simulink model "einspurmodell"  (R2017a)
settings: Solver=ode5  StartTime=0.0  StopTime=t_final  FixedStep=delta_t  RelTol=1e-3  EnableMultiTasking=on
PreLoadFcn:
  | model_preload_function;
InitFcn:
  | model_init_function;
values from neighbouring files (symbols this model uses):
  A = 1.9    [model_preload_function.m]
  alpha_q0 = pq_1*pq_2 + pq_1*pq_3 + pq_2*pq_3    (= 135)    [model_preload_function.m]
  alpha_q1 = -1 * (pq_1 + pq_2 + pq_3)    (= 23)    [model_preload_function.m]
  alpha_q_ = -1 * pq_1 * pq_2 * pq_3    (= 225)    [model_preload_function.m]
  c_h = 100000    [model_preload_function.m]
  c_v = 100000    [model_preload_function.m]
  c_w = 0.28    [model_preload_function.m]
  kiv = pv_1*pv_2    (= 0.48)    [model_preload_function.m]
  kpv = -pv_1-pv_2    (= 4.9)    [model_preload_function.m]
  l_h = 1.45    [model_preload_function.m]
  l_l0 = 10    [model_preload_function.m]
  l_v = 1.3    [model_preload_function.m]
  m = 1450    [model_preload_function.m]
  psi_0 = 0    [model_preload_function.m]
  rho_luft = 1.204    [model_preload_function.m]
  theta = 1920    [model_preload_function.m]
  v_0 = 10    [model_preload_function.m]
  v_soll = 10    [model_preload_function.m]
  w_ltr = 0    [model_preload_function.m]
  x_0 = 00    (= 0)    [model_preload_function.m]
  y_0 = 1.5    [model_preload_function.m]
undefined symbols (not defined in the file or in its folder): Ap, Bp, Cp, Dp
libraries: simulink x1
settings Model: Creator=piwi  LastModifiedBy=hi
settings DataIOCC: LimitDataPoints=on  SaveFormat=Array  SignalLoggingSaveFormat=ModelDataLogs  SignalLoggingName=sigsOut
settings OptimizationCC: LifeSpan=inf
settings DebuggingCC: SaveWithParameterizedLinksMsg=none  UnderspecifiedInitializationDetection=Classic  MergeDetectMultiDrivingBlocksExec=none  SignalResolutionControl=TryResolveAllWithWarning  MultiTaskDSMMsg=warning  MultiTaskCondExecSysMsg=none  SFUnexpectedBacktrackingDiag=warning  SFNoUnconditionalDefaultTransitionDiag=warning  SFExecutionAtInitializationDiag=none
settings HardwareCC: ProdBitPerPointer=32  ProdBitPerSizeT=32  ProdBitPerPtrDiffT=32  ProdLargestAtomicFloat=None  ProdIntDivRoundTo=Undefined  ProdEndianess=Unspecified  ProdWordSize=32  ProdHWDeviceType=32-bit Generic  TargetUnknown=on
settings ModelReferenceCC: PropagateSignalLabelsOutOfModel=off
settings GRTTargetCC: TargetLangStandard=C89/C90 (ANSI)  GeneratePreprocessorConditionals=Disable all  CombineOutputUpdateFcns=off  GRTInterface=on
settings ConfigComp: CovMetricSettings=dw  CovHtmlReporting=on  CovSaveCumulativeToWorkspaceVar=on  CovSaveSingleToWorkspaceVar=on  CovExternalEMLEnable=off

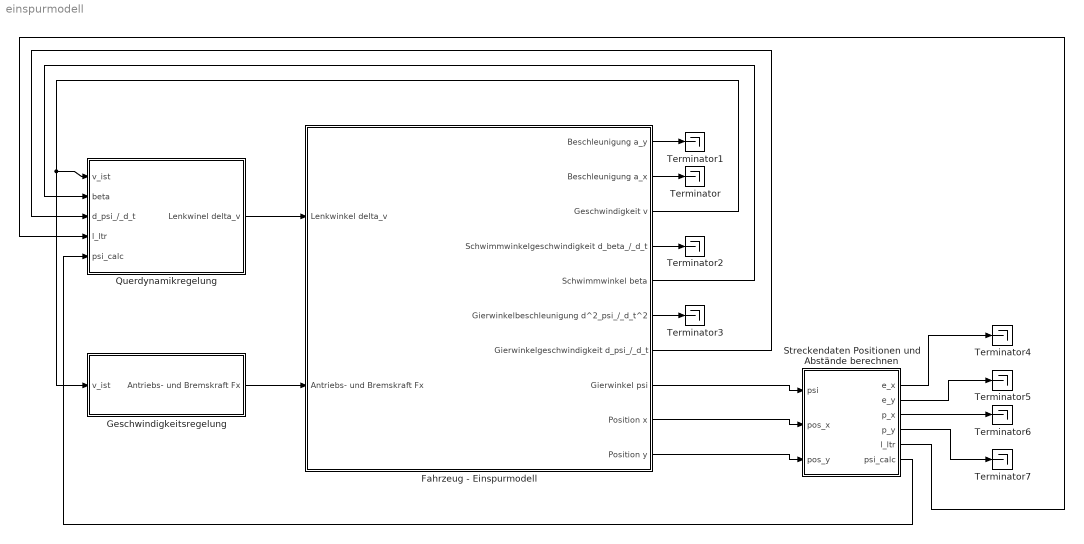
== system einspurmodell ==
  Fahrzeug - Einspurmodell : Subsystem
  Geschwindigkeitsregelung : Subsystem
  Querdynamikregelung : Subsystem
  Streckendaten Positionen und Abstände berechnen : Subsystem
  Terminator{,1..7} (8 alike) : Terminator
  wires:
  Fahrzeug - Einspurmodell/6(Gierwinkelbeschleunigung d^2_psi_/_d_t^2) -> Terminator3/1
  Fahrzeug - Einspurmodell/9(Position x) -> Streckendaten Positionen und Abstände berechnen/2(pos_x)
  Fahrzeug - Einspurmodell/10(Position y) -> Streckendaten Positionen und Abstände berechnen/3(pos_y)
  Fahrzeug - Einspurmodell/2(Beschleunigung a_x) -> Terminator/1
  Fahrzeug - Einspurmodell/1(Beschleunigung a_y) -> Terminator1/1
  Fahrzeug - Einspurmodell/4(Schwimmwinkelgeschwindigkeit d_beta_/_d_t) -> Terminator2/1
  Fahrzeug - Einspurmodell/8(Gierwinkel psi) -> Streckendaten Positionen und Abstände berechnen/1(psi)
  Streckendaten Positionen und Abstände berechnen/5(l_ltr) -> Querdynamikregelung/4(l_ltr)
  Streckendaten Positionen und Abstände berechnen/1(e_x) -> Terminator4/1
  Streckendaten Positionen und Abstände berechnen/2(e_y) -> Terminator5/1
  Streckendaten Positionen und Abstände berechnen/3(p_x) -> Terminator6/1
  Streckendaten Positionen und Abstände berechnen/4(p_y) -> Terminator7/1
  Fahrzeug - Einspurmodell/3(Geschwindigkeit v) -> Geschwindigkeitsregelung/1(v_ist), Querdynamikregelung/1(v_ist)
  Fahrzeug - Einspurmodell/5(Schwimmwinkel beta) -> Querdynamikregelung/2(beta)
  Fahrzeug - Einspurmodell/7(Gierwinkelgeschwindigkeit d_psi_/_d_t) -> Querdynamikregelung/3(d_psi_/_d_t)
  Querdynamikregelung/1(Lenkwinel delta_v) -> Fahrzeug - Einspurmodell/1(Lenkwinkel delta_v)
  Geschwindigkeitsregelung/1(Antriebs- und Bremskraft Fx) -> Fahrzeug - Einspurmodell/2(Antriebs- und Bremskraft Fx)
  Streckendaten Positionen und Abstände berechnen/6(psi_calc) -> Querdynamikregelung/5(psi_calc)

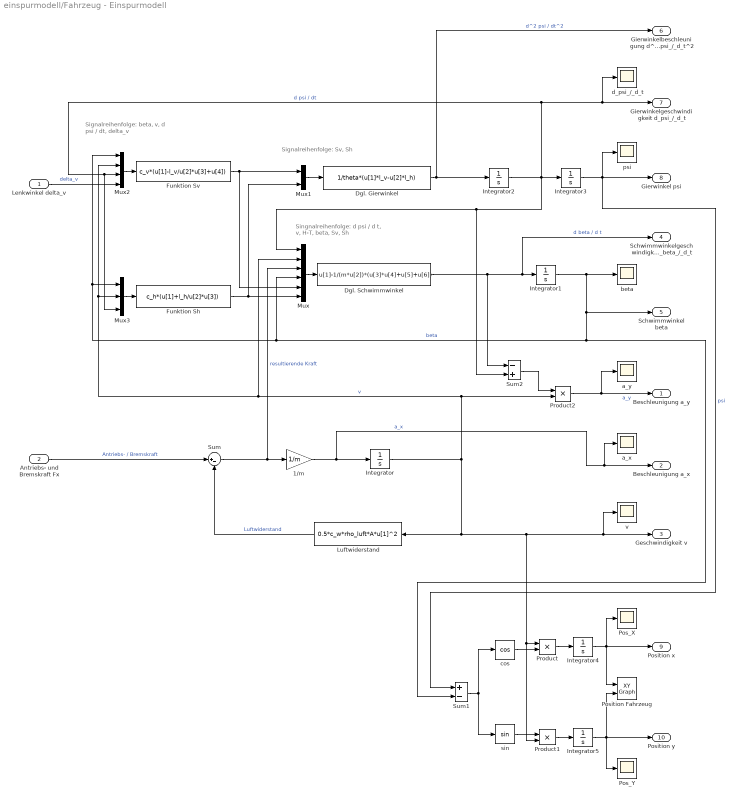
== system einspurmodell/Fahrzeug - Einspurmodell ==
  note: Singnalreihenfolge:
      | d psi / d t, v, H-T, beta, Sv, Sh
  note: Signalreihenfolge:
      | Sv, Sh
  note: Signalreihenfolge:
      | beta, v, d psi / dt, delta_v
  Lenkwinkel delta_v : Inport
  Antriebs- und Bremskraft Fx : Inport  Port=2
  1/m : Gain  Gain=1/m  SaturateOnIntegerOverflow=on  OutDataTypeStr=Inherit: Same as input  ParamDataTypeStr=Inherit: Same as input
  Dgl. Gierwinkel : Fcn  Expr=1/theta*(u[1]*l_v-u[2]*l_h)
  Dgl. Schwimmwinkel : Fcn  Expr=u[1]-1/(m*u[2])*(u[3]*u[4]+u[5]+u[6])
  Funktion Sh : Fcn  Expr=c_h*(u[1]+l_h/u[2]*u[3])
  Funktion Sv : Fcn  Expr=c_v*(u[1]-l_v/u[2]*u[3]+u[4])
  Integrator : Integrator  InitialCondition=v_0
  Integrator1 : Integrator
  Integrator2 : Integrator
  Integrator3 : Integrator  InitialCondition=psi_0
  Integrator4 : Integrator  InitialCondition=x_0
  Integrator5 : Integrator  InitialCondition=y_0
  Luftwiderstand : Fcn  Expr=0.5*c_w*rho_luft*A*u[1]^2
  Mux : Mux  Inputs=6
  Mux1 : Mux  Inputs=2
  Mux2 : Mux
  Mux3 : Mux  Inputs=3
  Pos_X : Scope
  Pos_Y : Scope
  Position Fahrzeug : simulink/Sinks/XY Graph  xmin=-50  xmax=600  ymin=-50  ymax=800  st=-1
  Product : Product  SaturateOnIntegerOverflow=on  OutDataTypeStr=Inherit: Same as first input
  Product1 : Product  SaturateOnIntegerOverflow=on  OutDataTypeStr=Inherit: Same as first input
  Product2 : Product  SaturateOnIntegerOverflow=on  OutDataTypeStr=Inherit: Same as first input
  Sum : Sum  Inputs=|+-  SaturateOnIntegerOverflow=on
  Sum1 : Sum  Inputs=+-  SaturateOnIntegerOverflow=on
  Sum2 : Sum  Inputs=-+  SaturateOnIntegerOverflow=on
  a_x : Scope
  a_y : Scope
  beta : Scope
  cos : Trigonometry  Operator=cos
  d_psi_/_d_t : Scope
  psi : Scope
  sin : Trigonometry
  v : Scope
  Beschleunigung a_y : Outport
  Beschleunigung a_x : Outport  Port=2
  Geschwindigkeit v : Outport  Port=3
  Schwimmwinkelgeschwindigkeit d_beta_/_d_t : Outport  Port=4
  Schwimmwinkel beta : Outport  Port=5
  Gierwinkelbeschleunigung d^2_psi_/_d_t^2 : Outport  Port=6
  Gierwinkelgeschwindigkeit d_psi_/_d_t : Outport  Port=7
  Gierwinkel psi : Outport  Port=8
  Position x : Outport  Port=9
  Position y : Outport  Port=10
  wires:
  Sum/1 -> 1/m/1, Mux/3  "resultierende Kraft"
  1/m/1 -> Integrator/1, a_x/1, Beschleunigung a_x/1  "a_x"
  Integrator/1 -> Luftwiderstand/1, Product1/2, Product/1, Geschwindigkeit v/1, v/1, Mux/2, Mux2/2, Mux3/2, Product2/2  "v"
  Luftwiderstand/1 -> Sum/2  "Luftwiderstand"
  Antriebs- und Bremskraft Fx/1 -> Sum/1  "Antriebs- / Bremskraft"
  Mux/1 -> Dgl. Schwimmwinkel/1
  Integrator1/1 -> Mux/4, Mux2/1, Mux3/1, Sum1/2, Schwimmwinkel beta/1, beta/1  "beta"
  Dgl. Schwimmwinkel/1 -> Schwimmwinkelgeschwindigkeit d_beta_/_d_t/1, Integrator1/1, Sum2/1  "d beta / d t"
  Dgl. Gierwinkel/1 -> Integrator2/1, Gierwinkelbeschleunigung d^2_psi_/_d_t^2/1  "d^2 psi / dt^2"
  Integrator2/1 -> Sum2/2, Mux/1, Mux3/3, Mux2/3, d_psi_/_d_t/1, Gierwinkelgeschwindigkeit d_psi_/_d_t/1, Integrator3/1  "d psi / dt"
  Mux1/1 -> Dgl. Gierwinkel/1
  Integrator3/1 -> Sum1/1, Gierwinkel psi/1, psi/1  "psi"
  Sum1/1 -> cos/1, sin/1
  Mux2/1 -> Funktion Sv/1
  Mux3/1 -> Funktion Sh/1
  Lenkwinkel delta_v/1 -> Mux2/4  "delta_v"
  Funktion Sh/1 -> Mux1/2, Mux/6
  Funktion Sv/1 -> Mux/5, Mux1/1
  Product/1 -> Integrator4/1
  Product1/1 -> Integrator5/1
  sin/1 -> Product1/1
  Product2/1 -> Beschleunigung a_y/1, a_y/1  "a_y"
  Sum2/1 -> Product2/1
  Integrator4/1 -> Pos_X/1, Position x/1, Position Fahrzeug/1
  Integrator5/1 -> Pos_Y/1, Position y/1, Position Fahrzeug/2
  cos/1 -> Product/2

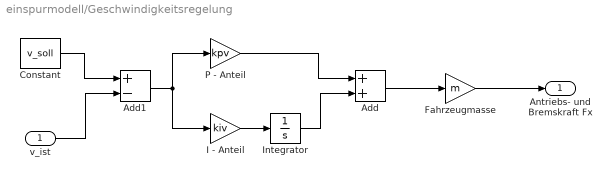
== system einspurmodell/Geschwindigkeitsregelung ==
  v_ist : Inport
  Add : Sum
  Add1 : Sum  Inputs=+-
  Constant : Constant  Value=v_soll
  Fahrzeugmasse : Gain  Gain=m
  I - Anteil : Gain  Gain=kiv
  Integrator : Integrator
  P - Anteil : Gain  Gain=kpv
  Antriebs- und Bremskraft Fx : Outport
  wires:
  Add1/1 -> I - Anteil/1, P - Anteil/1
  Add/1 -> Fahrzeugmasse/1
  Integrator/1 -> Add/2
  Constant/1 -> Add1/1
  I - Anteil/1 -> Integrator/1
  P - Anteil/1 -> Add/1
  Fahrzeugmasse/1 -> Antriebs- und Bremskraft Fx/1
  v_ist/1 -> Add1/2

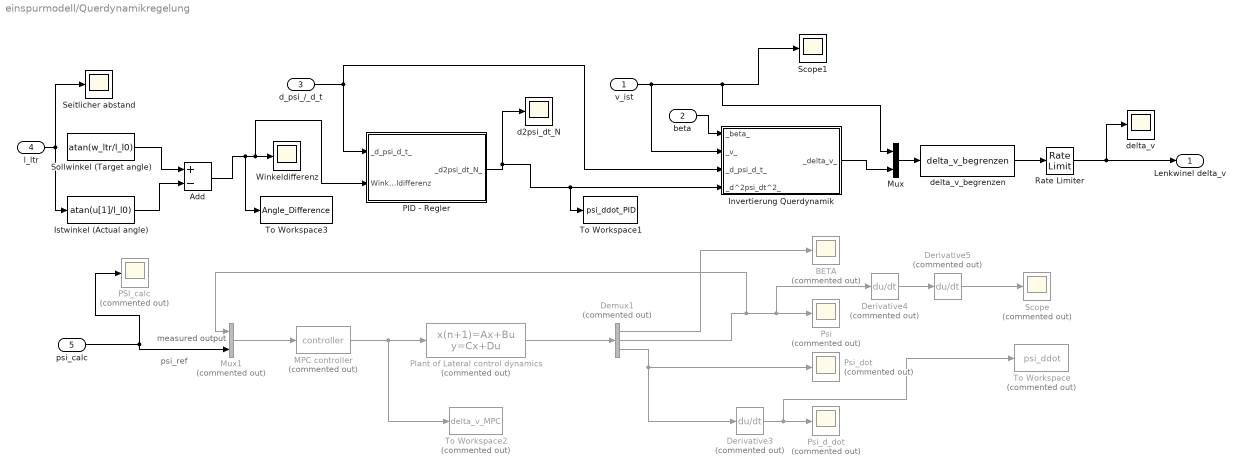
== system einspurmodell/Querdynamikregelung ==
  note: measured
      | output
  note: psi_ref
  v_ist : Inport
  beta : Inport  Port=2
  d_psi_/_d_t : Inport  Port=3
  l_ltr : Inport  Port=4
  psi_calc : Inport  Port=5
  Add : Sum  Inputs=+-
  BETA : Scope  Commented=on
  Demux1 : Demux  Commented=on  Outputs=3
  Derivative3 : Derivative  Commented=on
  Derivative4 : Derivative  Commented=on
  Derivative5 : Derivative  Commented=on
  Invertierung Querdynamik : Subsystem
  "Istwinkel (Actual angle) " : Fcn  Expr=atan(u[1]/l_l0)
  MPC controller : S-Function  Commented=on  FunctionName=controller  SFunctionDeploymentMode=off  EnableBusSupport=off
  Mux : Mux  Inputs=2
  Mux1 : Mux  Commented=on  Inputs=2
  PID - Regler : Subsystem
  PSI_calc : Scope  Commented=on
  Plant of Lateral control dynamics : DiscreteStateSpace  Commented=on  A=Ap  B=Bp  C=Cp  D=Dp  SampleTime=-1
  Psi : Scope  Commented=on
  Psi_d_dot : Scope  Commented=on
  Psi_dot : Scope  Commented=on
  Rate Limiter : RateLimiter  RisingSlewLimit=0.5  FallingSlewLimit=-0.5
  Scope : Scope  Commented=on
  Scope1 : Scope
  Seitlicher abstand : Scope
  Sollwinkel (Target angle) : Constant  Value=atan(w_ltr/l_l0)
  To Workspace : ToWorkspace  Commented=on  VariableName=psi_ddot  SaveFormat=Structure With Time  SampleTime=-1
  To Workspace1 : ToWorkspace  VariableName=psi_ddot_PID  SaveFormat=Structure With Time  SampleTime=-1
  To Workspace2 : ToWorkspace  Commented=on  VariableName=delta_v_MPC  SaveFormat=Structure With Time  SampleTime=-1
  To Workspace3 : ToWorkspace  VariableName=Angle_Difference  SaveFormat=Structure With Time  SampleTime=-1
  Winkeldifferenz : Scope
  d2psi_dt_N : Scope
  delta_v : Scope
  delta_v_begrenzen : S-Function  FunctionName=delta_v_begrenzen  SFunctionDeploymentMode=off  EnableBusSupport=off
  Lenkwinel delta_v : Outport
  wires:
  Rate Limiter/1 -> Lenkwinel delta_v/1, delta_v/1
  v_ist/1 -> Invertierung Querdynamik/2(_v_), Mux/1, Scope1/1
  d_psi_/_d_t/1 -> Invertierung Querdynamik/3(_d_psi_d_t_), PID - Regler/1(_d_psi_d_t_)
  Mux/1 -> delta_v_begrenzen/1
  Invertierung Querdynamik/1(_delta_v_) -> Mux/2
  delta_v_begrenzen/1 -> Rate Limiter/1
  Add/1 -> PID - Regler/2(Winkeldifferenz), Winkeldifferenz/1, To Workspace3/1
  Sollwinkel (Target angle)/1 -> Add/1
  l_ltr/1 -> Seitlicher abstand/1, "Istwinkel (Actual angle) "/1
  PID - Regler/1(_d2psi_dt_N_) -> To Workspace1/1, Invertierung Querdynamik/4(_d^2psi_dt^2_), d2psi_dt_N/1
  psi_calc/1 -> Mux1/2, PSI_calc/1
  beta/1 -> Invertierung Querdynamik/1(_beta_)
  "Istwinkel (Actual angle) "/1 -> Add/2
  Plant of Lateral control dynamics/1 -> Demux1/1
  Demux1/1 -> BETA/1
  Demux1/2 -> Derivative4/1, Psi/1, Mux1/1
  Demux1/3 -> Psi_dot/1, Derivative3/1
  Derivative3/1 -> Psi_d_dot/1, To Workspace/1
  Derivative4/1 -> Derivative5/1
  Derivative5/1 -> Scope/1
  Mux1/1 -> MPC controller/1
  MPC controller/1 -> To Workspace2/1, Plant of Lateral control dynamics/1

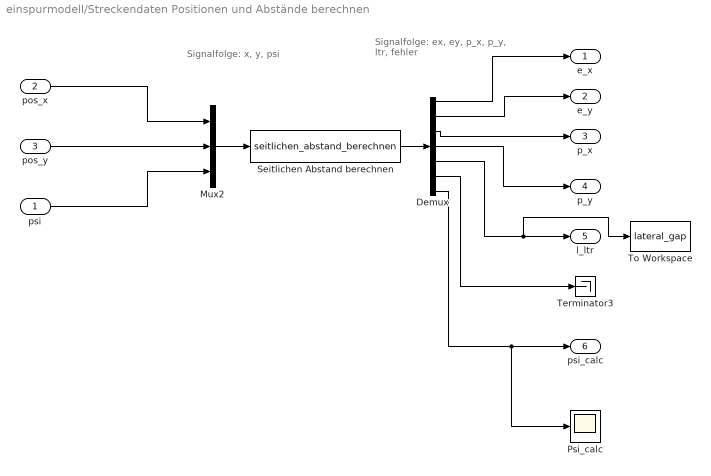
== system einspurmodell/Streckendaten Positionen und Abstände berechnen ==
  note: Signalfolge:
      | ex, ey, p_x, p_y, ltr, fehler
  note: Signalfolge:
      | x, y, psi
  psi : Inport
  pos_x : Inport  Port=2
  pos_y : Inport  Port=3
  Demux : Demux  Outputs=7
  Mux2 : Mux  Inputs=3
  Psi_calc : Scope
  Seitlichen Abstand berechnen : S-Function  FunctionName=seitlichen_abstand_berechnen  SFunctionDeploymentMode=off  EnableBusSupport=off
  Terminator3 : Terminator
  To Workspace : ToWorkspace  VariableName=lateral_gap  SaveFormat=Structure With Time  SampleTime=-1
  e_x : Outport
  e_y : Outport  Port=2
  p_x : Outport  Port=3
  p_y : Outport  Port=4
  l_ltr : Outport  Port=5
  psi_calc : Outport  Port=6
  wires:
  psi/1 -> Mux2/3
  Mux2/1 -> Seitlichen Abstand berechnen/1
  Seitlichen Abstand berechnen/1 -> Demux/1
  Demux/1 -> e_x/1
  Demux/2 -> e_y/1
  pos_x/1 -> Mux2/1
  pos_y/1 -> Mux2/2
  Demux/3 -> p_x/1
  Demux/4 -> p_y/1
  Demux/5 -> To Workspace/1, l_ltr/1
  Demux/6 -> Terminator3/1
  Demux/7 -> Psi_calc/1, psi_calc/1

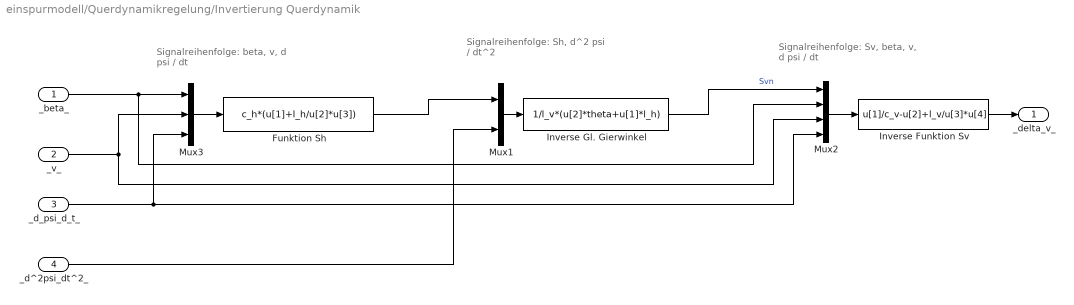
== system einspurmodell/Querdynamikregelung/Invertierung Querdynamik ==
  note: Signalreihenfolge:
      | Sv, beta, v, d psi / dt
  note: Signalreihenfolge:
      | beta, v, d psi / dt
  note: Signalreihenfolge:
      | Sh, d^2 psi / dt^2
  _beta_ : Inport
  _v_ : Inport  Port=2
  _d_psi_d_t_ : Inport  Port=3
  _d^2psi_dt^2_ : Inport  Port=4
  Funktion Sh : Fcn  Expr=c_h*(u[1]+l_h/u[2]*u[3])
  Inverse Funktion Sv : Fcn  Expr=u[1]/c_v-u[2]+l_v/u[3]*u[4]
  Inverse Gl. Gierwinkel : Fcn  Expr=1/l_v*(u[2]*theta+u[1]*l_h)
  Mux1 : Mux  Inputs=2
  Mux2 : Mux
  Mux3 : Mux  Inputs=3
  _delta_v_ : Outport
  wires:
  Mux2/1 -> Inverse Funktion Sv/1
  Inverse Gl. Gierwinkel/1 -> Mux2/1  "Svn"
  Mux1/1 -> Inverse Gl. Gierwinkel/1
  Mux3/1 -> Funktion Sh/1
  Funktion Sh/1 -> Mux1/1
  Inverse Funktion Sv/1 -> _delta_v_/1
  _d^2psi_dt^2_/1 -> Mux1/2
  _d_psi_d_t_/1 -> Mux3/3, Mux2/4
  _beta_/1 -> Mux3/1, Mux2/2
  _v_/1 -> Mux3/2, Mux2/3

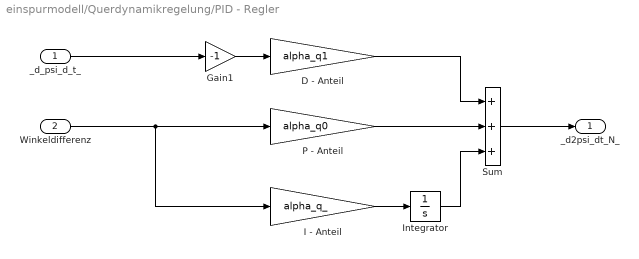
== system einspurmodell/Querdynamikregelung/PID - Regler ==
  _d_psi_d_t_ : Inport
  Winkeldifferenz : Inport  Port=2
  D - Anteil : Gain  Gain=alpha_q1  SaturateOnIntegerOverflow=on  OutDataTypeStr=Inherit: Same as input  ParamDataTypeStr=Inherit: Same as input
  Gain1 : Gain  Gain=-1  SaturateOnIntegerOverflow=on  OutDataTypeStr=Inherit: Same as input  ParamDataTypeStr=Inherit: Same as input
  I - Anteil : Gain  Gain=alpha_q_  SaturateOnIntegerOverflow=on  OutDataTypeStr=Inherit: Same as input  ParamDataTypeStr=Inherit: Same as input
  Integrator : Integrator
  P - Anteil : Gain  Gain=alpha_q0  SaturateOnIntegerOverflow=on  OutDataTypeStr=Inherit: Same as input  ParamDataTypeStr=Inherit: Same as input
  Sum : Sum  Inputs=+++  SaturateOnIntegerOverflow=on
  _d2psi_dt_N_ : Outport
  wires:
  P - Anteil/1 -> Sum/2
  Sum/1 -> _d2psi_dt_N_/1
  D - Anteil/1 -> Sum/1
  I - Anteil/1 -> Integrator/1
  Gain1/1 -> D - Anteil/1
  Integrator/1 -> Sum/3
  Winkeldifferenz/1 -> I - Anteil/1, P - Anteil/1
  _d_psi_d_t_/1 -> Gain1/1
